simulink library "ModC_Planner"  (R2018a)
settings: Solver=VariableStepAuto  StartTime=0.0  StopTime=10.0  RelTol=1e-3
settings Model: Creator=Lisandro Cocca  LastModifiedBy=Lisandro Cocca

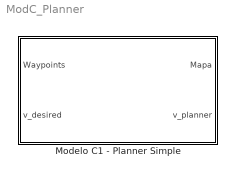
== system ModC_Planner ==
  Modelo C1 - Planner Simple : Subsystem

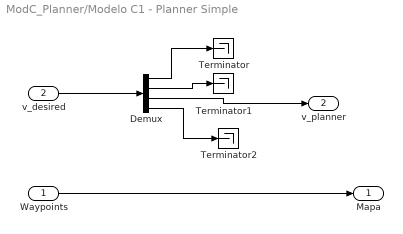
== system ModC_Planner/Modelo C1 - Planner Simple ==
  Waypoints : Inport
  v_desired : Inport  Port=2
  Demux : Demux
  Terminator : Terminator
  Terminator1 : Terminator
  Terminator2 : Terminator
  Mapa : Outport
  v_planner : Outport  Port=2
  wires:
  Waypoints/1 -> Mapa/1
  v_desired/1 -> Demux/1
  Demux/3 -> v_planner/1
  Demux/1 -> Terminator/1
  Demux/2 -> Terminator1/1
  Demux/4 -> Terminator2/1
